simulink model "powergain1"  (R2023a)
settings: Solver=VariableStepAuto  StartTime=0.0  StopTime=10.0  RelTol=1e-3
settings Model: Creator=desire  LastModifiedBy=desire

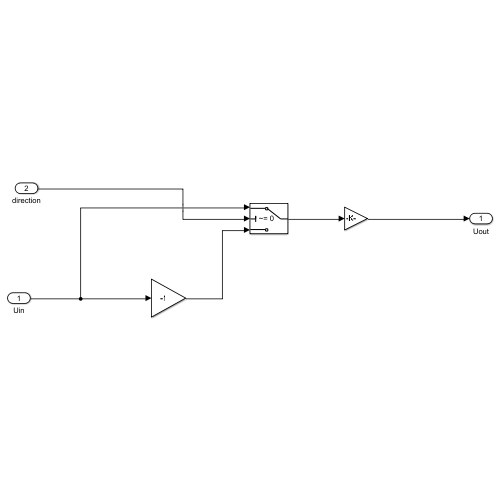
[thumbnail: Simulink's stored preview of the top-level diagram]
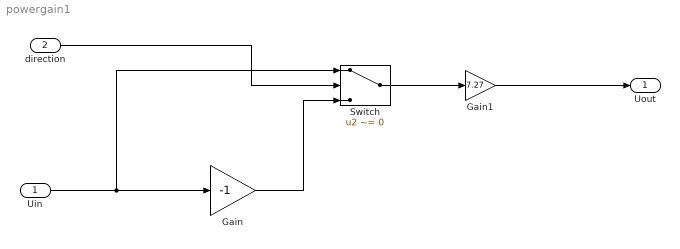
== system powergain1 ==
  Uin : Inport  OutMin=[0]  OutMax=[3.3]
  direction : Inport  Port=2
  Gain : Gain  Gain=-1
  Gain1 : Gain  Gain=7.27
  Switch : Switch  Criteria=u2 ~= 0  SaturateOnIntegerOverflow=off  InputSameDT=off
  Uout : Outport  OutMin=[0]  OutMax=[24]
  wires:
  direction/1 -> Switch/2
  Uin/1 -> Switch/1, Gain/1
  Gain/1 -> Switch/3
  Switch/1 -> Gain1/1
  Gain1/1 -> Uout/1
